simulink model "powertrain"  (R2024b)
settings: Solver=VariableStepAuto  StartTime=0.0  StopTime=10.0  RelTol=1e-3
model workspace (MAT data in the model file):
  eta_gearbox = 0.98
  eta_inverter = 1
(part 1 of 4)
settings Model: Creator=account  LastModifiedBy=account

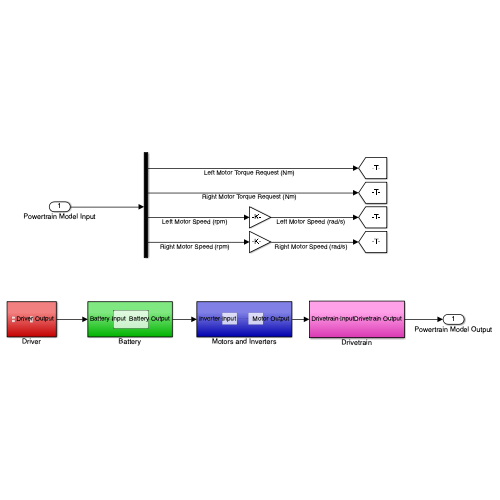
[thumbnail: Simulink's stored preview of the top-level diagram]
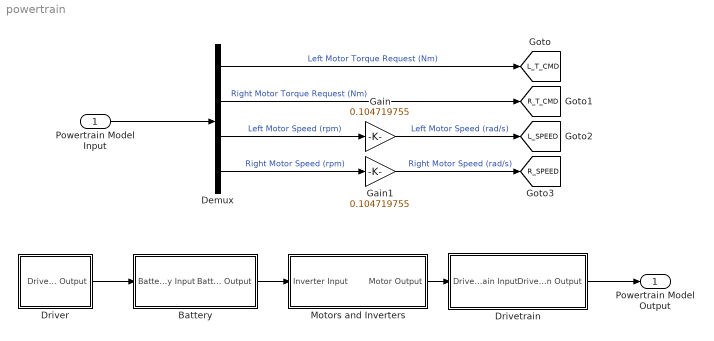
== system powertrain ==
  Powertrain Model Input : Inport
  Battery : Subsystem
  Demux : Demux
  Driver : Subsystem
  Drivetrain : Subsystem
  Gain : Gain  Gain=0.104719755
  Gain1 : Gain  Gain=0.104719755
  Motors and Inverters : Subsystem
  Powertrain Model Output : Outport
  tag scope: L_SPEED=global, L_T_CMD=global, R_SPEED=global, R_T_CMD=global
  wires:
  Motors and Inverters/1(Motor Output) -> Drivetrain/1(Drivetrain Input)
  Battery/1(Battery Output) -> Motors and Inverters/1(Inverter Input)
  Driver/1(Driver Output) -> Battery/1(Battery Input)
  Drivetrain/1(Drivetrain Output) -> Powertrain Model Output/1
  Powertrain Model Input/1 -> Demux/1
  Demux/1 -> [L_T_CMD]  "Left Motor Torque Request (Nm)"
  Demux/2 -> [R_T_CMD]  "Right Motor Torque Request (Nm)"
  Demux/3 -> Gain/1  "Left Motor Speed (rpm)"
  Demux/4 -> Gain1/1  "Right Motor Speed (rpm)"
  Gain/1 -> [L_SPEED]  "Left Motor Speed (rad/s)"
  Gain1/1 -> [R_SPEED]  "Right Motor Speed (rad/s)"

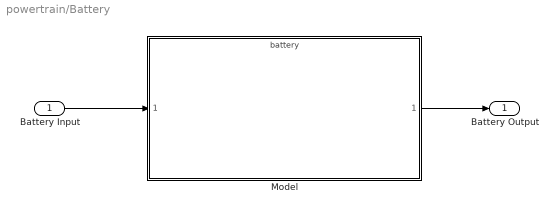
== system powertrain/Battery ==
  Battery Input : Inport
  Model : ModelReference  ModelNameDialog=battery.slx  SimulationMode=Normal  ModelReferenceVersion=1.8
  Battery Output : Outport
  wires:
  Battery Input/1 -> Model/1
  Model/1 -> Battery Output/1

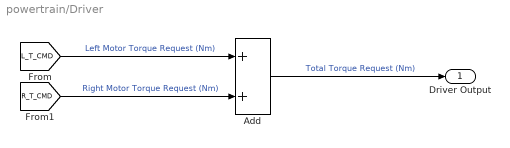
== system powertrain/Driver ==
  Add : Sum
  Driver Output : Outport
  wires:
  Add/1 -> Driver Output/1  "Total Torque Request (Nm)"
  [L_T_CMD] -> Add/1  "Left Motor Torque Request (Nm)"
  [R_T_CMD] -> Add/2  "Right Motor Torque Request (Nm)"

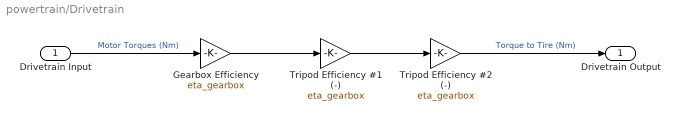
== system powertrain/Drivetrain ==
  Drivetrain Input : Inport
  Gearbox Efficiency : Gain  Gain=eta_gearbox
  Tripod Efficiency #1 (-) : Gain  Gain=eta_gearbox
  Tripod Efficiency #2 (-) : Gain  Gain=eta_gearbox
  Drivetrain Output : Outport
  wires:
  Drivetrain Input/1 -> Gearbox Efficiency/1  "Motor Torques (Nm)"
  Gearbox Efficiency/1 -> Tripod Efficiency #1 (-)/1
  Tripod Efficiency #1 (-)/1 -> Tripod Efficiency #2 (-)/1
  Tripod Efficiency #2 (-)/1 -> Drivetrain Output/1  "Torque to Tire (Nm)"

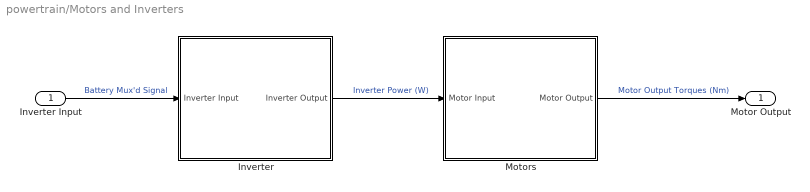
== system powertrain/Motors and Inverters ==
  Inverter Input : Inport
  Inverter : Subsystem
  Motors : Subsystem
  Motor Output : Outport
  wires:
  Inverter Input/1 -> Inverter/1(Inverter Input)  "Battery Mux'd Signal"
  Inverter/1(Inverter Output) -> Motors/1(Motor Input)  "Inverter Power (W)"
  Motors/1(Motor Output) -> Motor Output/1  "Motor Output Torques (Nm)"

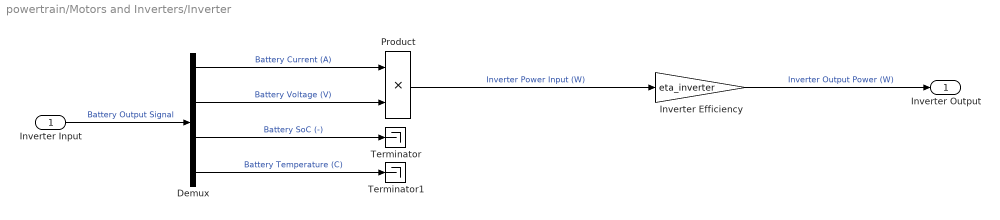
== system powertrain/Motors and Inverters/Inverter ==
  Inverter Input : Inport
  Demux : Demux
  Inverter Efficiency : Gain  Gain=eta_inverter
  Product : Product
  Terminator : Terminator
  Terminator1 : Terminator
  Inverter Output : Outport
  wires:
  Inverter Efficiency/1 -> Inverter Output/1  "Inverter Output Power (W)"
  Inverter Input/1 -> Demux/1  "Battery Output Signal"
  Demux/1 -> Product/1  "Battery Current (A)"
  Demux/2 -> Product/2  "Battery Voltage (V)"
  Product/1 -> Inverter Efficiency/1  "Inverter Power Input (W)"
  Demux/3 -> Terminator/1  "Battery SoC (-)"
  Demux/4 -> Terminator1/1  "Battery Temperature (C)"

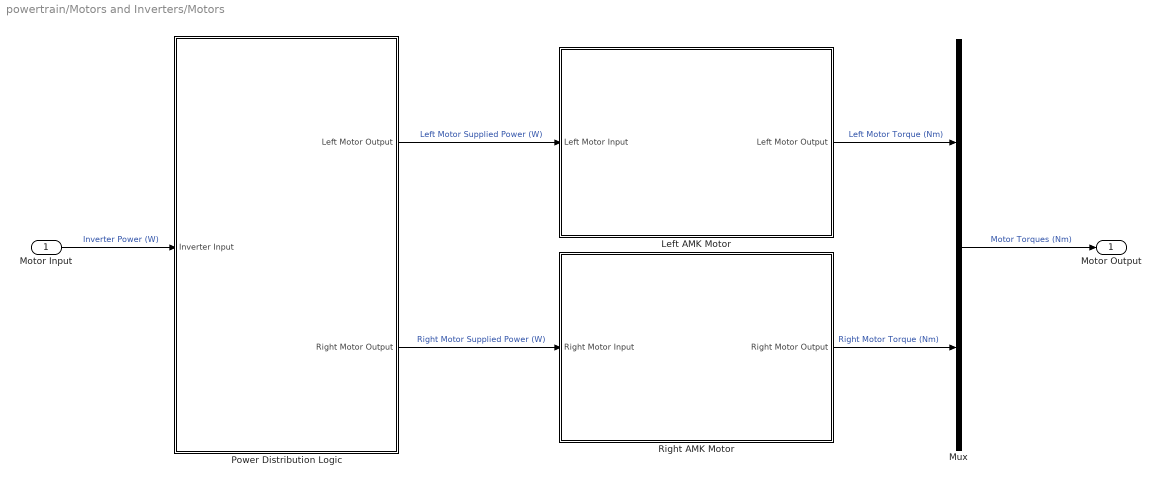
== system powertrain/Motors and Inverters/Motors ==
  Motor Input : Inport
  Left AMK Motor : Subsystem
  Mux : Mux  Inputs=2
  Power Distribution Logic : Subsystem
  Right AMK Motor : Subsystem
  Motor Output : Outport
  wires:
  Motor Input/1 -> Power Distribution Logic/1(Inverter Input)  "Inverter Power (W)"
  Power Distribution Logic/1(Left Motor Output) -> Left AMK Motor/1(Left Motor Input)  "Left Motor Supplied Power (W)"
  Power Distribution Logic/2(Right Motor Output) -> Right AMK Motor/1(Right Motor Input)  "Right Motor Supplied Power (W)"
  Left AMK Motor/1(Left Motor Output) -> Mux/1  "Left Motor Torque (Nm)"
  Right AMK Motor/1(Right Motor Output) -> Mux/2  "Right Motor Torque (Nm)"
  Mux/1 -> Motor Output/1  "Motor Torques (Nm)"
